simulink model "questionC"  (R2017b)
settings: Solver=VariableStepAuto  StartTime=0.0  StopTime=10.0  RelTol=1e-3
libraries: simulink x2, vrlib x2
settings Model: Creator=zephi  LastModifiedBy=kenny.nguyen

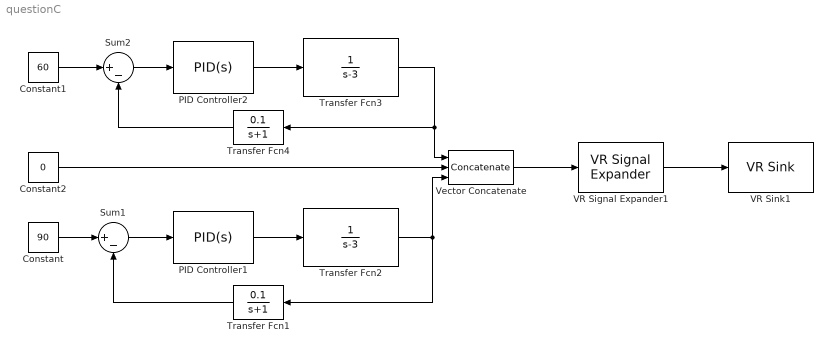
== system questionC ==
  Constant : Constant  Value=90
  Constant1 : Constant  Value=60
  Constant2 : Constant  Value=0
  PID Controller1 : simulink/Continuous/PID Controller  Controller=PID  TimeDomain=Continuous-time  SampleTime=-1  IntegratorMethod=Forward Euler  FilterMethod=Forward Euler  Form=Parallel  UseFilter=on  ControllerParametersSource=internal  P=12.6937617429655  I=5.12830595066741  D=6.24506148616122  N=16.1607937491403  InitialConditionSource=internal  InitialConditionForIntegrator=0  InitialConditionForFilter=0  ExternalReset=none  LimitOutput=on  UpperSaturationLimit=inf  LowerSaturationLimit=-inf  LinearizeAsGain=on  AntiWindupMode=none  Kb=1  TrackingMode=off  Kt=1  PParamMin=0  PParamMax=100  IParamMin=0  IParamMax=100  DParamMin=0  DParamMax=100  NParamMin=[]  NParamMax=[]  KbParamMin=[]  KbParamMax=[]  KtParamMin=[]  KtParamMax=[]  POutMin=2  POutMax=2  POutDataTypeStr=double  PGainOutDataTypeStr=double  PProdOutDataTypeStr=double  IOutMin=2  IOutMax=2  IOutDataTypeStr=double  IGainOutDataTypeStr=double  IProdOutDataTypeStr=double  DOutMin=2  DOutMax=2  DOutDataTypeStr=double  DGainOutDataTypeStr=double  DProdOutDataTypeStr=double  NOutMin=2  NOutMax=2  NOutDataTypeStr=double  NGainOutDataTypeStr=double  NProdOutDataTypeStr=double  KbOutMin=[]  KbOutMax=[]  KtOutMin=[]  KtOutMax=[]  IntegratorOutMin=[]  IntegratorOutMax=[]  FilterOutMin=[]  FilterOutMax=[]  SumOutMin=[]  SumOutMax=[]  SumI1OutMin=[]  SumI1OutMax=[]  SumI2OutMin=[]  SumI2OutMax=[]  SumI3OutMin=[]  SumI3OutMax=[]  SumDOutMin=[]  SumDOutMax=[]  SaturationOutMin=[]  SaturationOutMax=[]  IntegratorContinuousStateAttributes=''  IntegratorStateMustResolveToSignalObject=off  IntegratorRTWStateStorageClass=Auto  FilterContinuousStateAttributes=''  FilterStateMustResolveToSignalObject=off  FilterRTWStateStorageClass=Auto  DifferentiatorICPrevScaledInput=0  DifferentiatorOutMin=[]  DifferentiatorOutMax=[]  InitialConditionSetting=State (most efficient)  FilterDiffOutCoefMin=[]  FilterDiffOutCoefMax=[]  SumDenOutMin=[]  SumDenOutMax=[]  SumNumOutMin=[]  SumNumOutMax=[]  ReciprocalOutMin=[]  ReciprocalOutMax=[]  DivideOutMin=[]  DivideOutMax=[]  TunerSelectOption=Transfer Function Based (PID Tuner App)
  PID Controller2 : simulink/Continuous/PID Controller  Controller=PID  TimeDomain=Continuous-time  SampleTime=-1  IntegratorMethod=Forward Euler  FilterMethod=Forward Euler  Form=Parallel  UseFilter=on  ControllerParametersSource=internal  P=50.7923816882802  I=38.8831360917221  D=15.5897118066608  N=25.8047624023156  InitialConditionSource=internal  InitialConditionForIntegrator=0  InitialConditionForFilter=0  ExternalReset=none  LimitOutput=on  UpperSaturationLimit=inf  LowerSaturationLimit=-inf  LinearizeAsGain=on  AntiWindupMode=none  Kb=1  TrackingMode=off  Kt=1  PParamMin=0  PParamMax=100  IParamMin=0  IParamMax=100  DParamMin=0  DParamMax=100  NParamMin=[]  NParamMax=[]  KbParamMin=[]  KbParamMax=[]  KtParamMin=[]  KtParamMax=[]  POutMin=2  POutMax=2  POutDataTypeStr=double  PGainOutDataTypeStr=double  PProdOutDataTypeStr=double  IOutMin=2  IOutMax=2  IOutDataTypeStr=double  IGainOutDataTypeStr=double  IProdOutDataTypeStr=double  DOutMin=2  DOutMax=2  DOutDataTypeStr=double  DGainOutDataTypeStr=double  DProdOutDataTypeStr=double  NOutMin=2  NOutMax=2  NOutDataTypeStr=double  NGainOutDataTypeStr=double  NProdOutDataTypeStr=double  KbOutMin=[]  KbOutMax=[]  KtOutMin=[]  KtOutMax=[]  IntegratorOutMin=[]  IntegratorOutMax=[]  FilterOutMin=[]  FilterOutMax=[]  SumOutMin=[]  SumOutMax=[]  SumI1OutMin=[]  SumI1OutMax=[]  SumI2OutMin=[]  SumI2OutMax=[]  SumI3OutMin=[]  SumI3OutMax=[]  SumDOutMin=[]  SumDOutMax=[]  SaturationOutMin=[]  SaturationOutMax=[]  IntegratorContinuousStateAttributes=''  IntegratorStateMustResolveToSignalObject=off  IntegratorRTWStateStorageClass=Auto  FilterContinuousStateAttributes=''  FilterStateMustResolveToSignalObject=off  FilterRTWStateStorageClass=Auto  DifferentiatorICPrevScaledInput=0  DifferentiatorOutMin=[]  DifferentiatorOutMax=[]  InitialConditionSetting=State (most efficient)  FilterDiffOutCoefMin=[]  FilterDiffOutCoefMax=[]  SumDenOutMin=[]  SumDenOutMax=[]  SumNumOutMin=[]  SumNumOutMax=[]  ReciprocalOutMin=[]  ReciprocalOutMax=[]  DivideOutMin=[]  DivideOutMax=[]  TunerSelectOption=Transfer Function Based (PID Tuner App)
  Sum1 : Sum  Inputs=|+-  OutMin=2  OutMax=2
  Sum2 : Sum  Inputs=|+-  OutMin=2  OutMax=2
  Transfer Fcn1 : TransferFcn  Numerator=[0.1]  Denominator=[1 1]
  Transfer Fcn2 : TransferFcn  Denominator=[1 -3]
  Transfer Fcn3 : TransferFcn  Denominator=[1 -3]
  Transfer Fcn4 : TransferFcn  Numerator=[0.1]  Denominator=[1 1]
  VR Signal Expander1 : vrlib/VR Signal Expander  outwidth=4  outidx=[1 3 4]
      settings: SourceProductName=Simulink 3D Animation  SourceProductBaseCode=VR
  VR Sink1 : vrlib/VR Sink  InstantiateOnLoad=on  SampleTime=0.1  ViewEnable=on  RemoteChange=off  RemoteView=off  FieldsWritten=Axis.rotation.4.1.1.double  WorldFileName=telescope.wrl  WorldDescription=telescope  AutoView=on  VideoDimensions=[]  AllowVariableSize=off  FigureProperties="{'Position', 'Name', 'Viewpoint', 'CameraBound', 'CameraDirection', 'CameraPosition', 'CameraUpVector', 'ZoomFactor', 'Antialiasing', 'Headlight', 'Lighting', 'NavPanel', 'Sound', 'StatusBar', 'Stereo3D', 'Stereo3DCameraOffset', 'Stereo3DHIT', 'ToolBar', 'Textures', 'Transparency', 'Triad', 'Wireframe', 'NavZones', 'NavMode', 'NavSpeed', 'CaptureFileFormat', 'CaptureFileName', 'Record2DCompressMethod', 'Record2DCompressQuality', 'Record2D', 'Record2DFileName', 'Record2DFPS'; [5.0000000000000000e+00   9.2333333333333371e+01   7.7733333333333326e+02   4.7466666666666663e+02], 'telescope', '', 'on', [2.7185066862199242e-01   3.5298137558873295e-02  -9.6169187136767309e-01], [-1.3203721323728861e+00  -5.0383470414081233e-01   1.6952250900394183e+01], [-2.6588057115429577e-02   9.9922108972431511e-01   2.9159716544911580e-02], [1.0000000000000000e+00], 'on', 'on', 'on', 'halfbar', 'on', 'on', 'off', [1.0000000149011612e-01], [0.0000000000000000e+00], 'on', 'on', 'on', 'none', 'off', 'off', 'fly', 'normal', 'tif', '%f_anim_%n.tif', 'auto', [7.5000000000000000e+01], 'off', '%f_anim_%n.avi', 'auto'}"
      settings: SourceProductBaseCode=VR
  Vector Concatenate : Concatenate  NumInputs=3
  wires:
  Sum1/1 -> PID Controller1/1
  Transfer Fcn2/1 -> Transfer Fcn1/1, Vector Concatenate/3
  PID Controller1/1 -> Transfer Fcn2/1
  Constant/1 -> Sum1/1
  Vector Concatenate/1 -> VR Signal Expander1/1
  Transfer Fcn3/1 -> Vector Concatenate/1, Transfer Fcn4/1
  PID Controller2/1 -> Transfer Fcn3/1
  Constant1/1 -> Sum2/1
  Sum2/1 -> PID Controller2/1
  VR Signal Expander1/1 -> VR Sink1/1
  Constant2/1 -> Vector Concatenate/2
  Transfer Fcn4/1 -> Sum2/2
  Transfer Fcn1/1 -> Sum1/2
